simulink model "sim2"  (R2023a)
settings: Solver=VariableStepAuto  StartTime=0  StopTime=80  RelTol=1e-8
undefined symbols (not defined in the file or in its folder): K, T1, T2
settings Model: Creator=vasil  LastModifiedBy=vasil

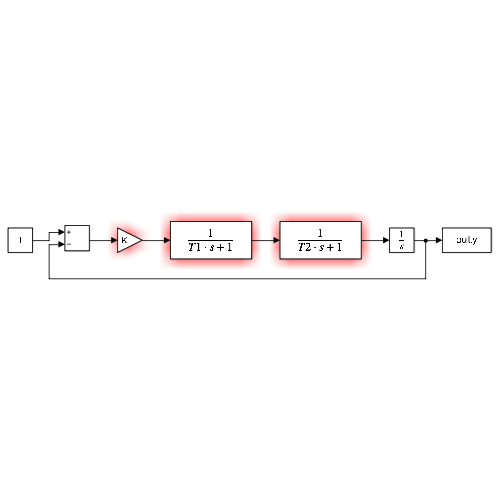
[thumbnail: Simulink's stored preview of the top-level diagram]
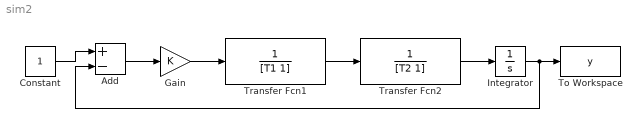
== system sim2 ==
  Add : Sum  Inputs=+-
  Constant : Constant
  Gain : Gain  Gain=K
  Integrator : Integrator
  To Workspace : ToWorkspace  VariableName=y  SaveFormat=Timeseries  SampleTime=-1
  Transfer Fcn1 : TransferFcn  Denominator=[T1 1]
  Transfer Fcn2 : TransferFcn  Denominator=[T2 1]
  wires:
  Constant/1 -> Add/1
  Add/1 -> Gain/1
  Transfer Fcn1/1 -> Transfer Fcn2/1
  Transfer Fcn2/1 -> Integrator/1
  Integrator/1 -> To Workspace/1, Add/2
  Gain/1 -> Transfer Fcn1/1
